simulink model "invertor"  (Simulink 8.3)
settings: Solver=ode45  StartTime=0.0  StopTime=0.5  RelTol=1e-3
libraries: powerlib x8, simulink x1, powerlib_meascontrol x1
settings Model: Creator=Singhal  LastModifiedBy=Singhal
settings OptimizationCC: ExpressionDepthLimit=2147483647
settings DebuggingCC: FcnCallInpInsideContextMsg=UseLocalSettings

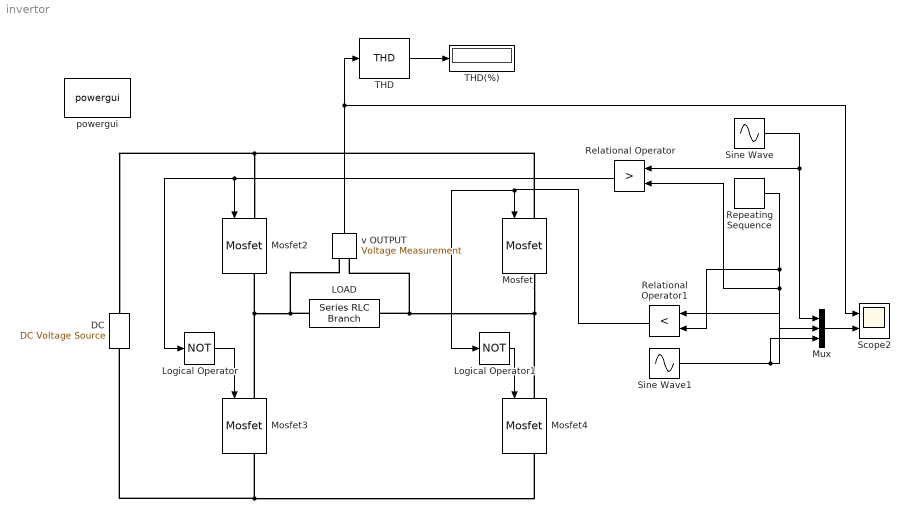
== system invertor ==
  DC : powerlib/Electrical Sources/DC Voltage Source  Amplitude=100  Measurements=None
  LOAD : powerlib/Elements/Series RLC Branch  LConnTagsString=__new0  RConnTagsString=__new0  BranchType=R  Resistance=20  Inductance=1e-3  SetiL0=off  InitialCurrent=0  Capacitance=1e-6  Setx0=off  InitialVoltage=0  Measurements=None
  Logical Operator : Logic  Operator=NOT  AllPortsSameDT=off  OutDataTypeStr=boolean
  Logical Operator1 : Logic  Operator=NOT  AllPortsSameDT=off  OutDataTypeStr=boolean
  Mosfet{,2..4} (4 alike) : powerlib/Power Electronics/Mosfet  Ron=0.1  Lon=0  Rd=0.01  Vfd=0  IC=0  Rs=1e5  Cs=inf  Measurements=on
  Mux : Mux  Inputs=3
  Relational Operator : RelationalOperator  Operator=>  OutDataTypeStr=boolean
  Relational Operator1 : RelationalOperator  Operator=<  OutDataTypeStr=boolean
  Repeating Sequence : simulink/Sources/Repeating Sequence  rep_seq_t=[0 0.005/20 0.01/20 0.015/20 0.02/20]  rep_seq_y=[0 10 0 -10 0]
  Scope2 : Scope  NumInputPorts=2
      settings: YMin=0~0  YMax=1~1  SaveName=ScopeData2
  Sine Wave : Sin  Amplitude=8  Frequency=50*2*3.14  SampleTime=0
  Sine Wave1 : Sin  Amplitude=8  Frequency=50*2*3.14  Phase=3.14  SampleTime=0
  THD : powerlib_meascontrol/Measurements/THD  Freq=60  Ts=0
  THD(%) : Display
  powergui : powerlib/powergui  Priority=1  SimulationMode=Discrete  SolverType=Tustin  SampleTime=50e-6  frequency=60  SPID=off  DisableSnubberDevices=off  DisableRonSwitches=off  DisableVfSwitches=off  SwTol=0  Interpol=off  DisplayEquations=off  Ts=0  methode=off  frequencyindice=0  Pbase=100e6  ErrMax=1e-4  Iterations=50  UnitsV=kV  UnitsW=MW  FunctionMessages=off  echomessages=off  HookPort=off  EnableUseOfTLC=off  x0status=blocks  RestoreLinks=warning  ResistiveCurrentMeasurement=off  Frange=[0:2:500]  Ylog=off  Xlog=on  ShowGrid=off  save=off  variable=ZData  structure=ScopeData  ZoomFFT=on  StartTime=0.0  cycles=1  DisplayStyle=2  fundamental=50  FreqAxis=off  MaxFrequency=1000  frequencyindicesteady=1  RmsSteady=1  display=off
  v OUTPUT : powerlib/Measurements/Voltage Measurement  PhasorSimulation=off  OutputType=Complex  PSBequivalent=0
  wires:
  v OUTPUT/1 -> Scope2/1, THD/1
  THD/1 -> THD(%)/1
  Sine Wave/1 -> Mux/1, Relational Operator/1
  Logical Operator/1 -> Mosfet3/1
  Repeating Sequence/1 -> Mux/2, Relational Operator/2, Relational Operator1/2
  Sine Wave1/1 -> Relational Operator1/1, Mux/3
  Logical Operator1/1 -> Mosfet4/1
  Relational Operator/1 -> Mosfet2/1, Logical Operator/1
  Relational Operator1/1 -> Logical Operator1/1, Mosfet/1
  Mux/1 -> Scope2/2
  connections:
  Mosfet/LConn1 -- DC/RConn1 -- Mosfet2/LConn1
  DC/LConn1 -- Mosfet3/RConn1 -- Mosfet4/RConn1
  Mosfet4/LConn1 -- Mosfet/RConn1 -- v OUTPUT/LConn2 -- LOAD/LConn1
  Mosfet3/LConn1 -- Mosfet2/RConn1 -- v OUTPUT/LConn1 -- LOAD/RConn1
